simulink model "closed_loop_rider_PID"  (R2018b)
settings: Solver=VariableStepAuto  StartTime=0.0  StopTime=17.3  RelTol=1e-3
values from neighbouring files (symbols this model uses):
  G11_den = bike_s.Denominator{1, 1}    [data_analysis.m]
  G11_num = bike_s.Numerator{1, 1}    [data_analysis.m]
  G12_den = bike_s.Denominator{1, 2}    [data_analysis.m]
  G12_num = bike_s.Numerator{1, 2}    [data_analysis.m]
  G21_den = bike_s.Denominator{2, 1}    [data_analysis.m]
  G21_num = bike_s.Numerator{2, 1}    [data_analysis.m]
  G22_den = bike_s.Denominator{2, 2}    [data_analysis.m]
  G22_num = bike_s.Numerator{2, 2}    [data_analysis.m]
libraries: simulink x2
settings Model: Creator=chris  LastModifiedBy=chris

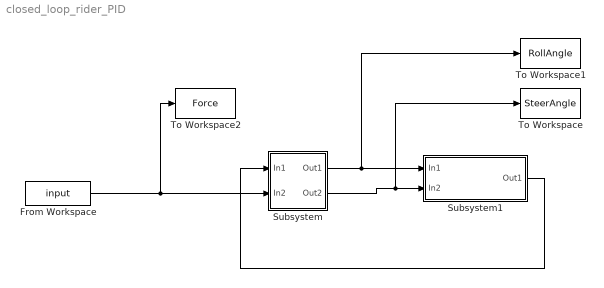
== system closed_loop_rider_PID ==
  From Workspace : FromWorkspace  VariableName=input  SampleTime=0
  Subsystem : Subsystem
  Subsystem1 : Subsystem
  To Workspace : ToWorkspace  VariableName=SteerAngle  SaveFormat=Timeseries  SampleTime=-1
  To Workspace1 : ToWorkspace  VariableName=RollAngle  SaveFormat=Timeseries  SampleTime=-1
  To Workspace2 : ToWorkspace  VariableName=Force  SaveFormat=Timeseries  SampleTime=-1
  wires:
  From Workspace/1 -> Subsystem/2(In2), To Workspace2/1
  Subsystem/1(Out1) -> To Workspace1/1, Subsystem1/1(In1)
  Subsystem1/1(Out1) -> Subsystem/1(In1)
  Subsystem/2(Out2) -> To Workspace/1, Subsystem1/2(In2)

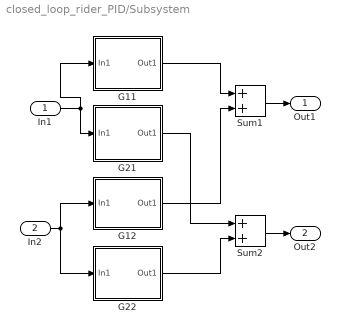
== system closed_loop_rider_PID/Subsystem ==
  In1 : Inport
  In2 : Inport  Port=2
  G11 : Subsystem
  G12 : Subsystem
  G21 : Subsystem
  G22 : Subsystem
  Sum1 : Sum  SaturateOnIntegerOverflow=on  InputSameDT=on  OutDataTypeStr=Inherit: Same as first input
  Sum2 : Sum  SaturateOnIntegerOverflow=on  InputSameDT=on  OutDataTypeStr=Inherit: Same as first input
  Out1 : Outport  InitialOutput=0
  Out2 : Outport  Port=2  InitialOutput=0
  wires:
  In1/1 -> G11/1(In1), G21/1(In1)
  G21/1(Out1) -> Sum2/1
  G12/1(Out1) -> Sum1/2
  G11/1(Out1) -> Sum1/1
  G22/1(Out1) -> Sum2/2
  In2/1 -> G12/1(In1), G22/1(In1)
  Sum1/1 -> Out1/1
  Sum2/1 -> Out2/1

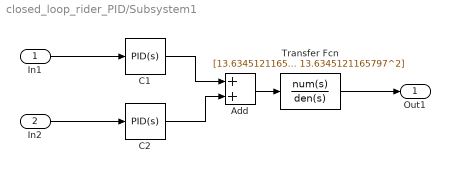
== system closed_loop_rider_PID/Subsystem1 ==
  In1 : Inport
  In2 : Inport  Port=2
  Add : Sum
  C1 : simulink/Continuous/PID Controller  Controller=PID  Form=Parallel  TimeDomain=Continuous-time  SampleTime=-1  IntegratorMethod=Forward Euler  FilterMethod=Forward Euler  ControllerParametersSource=internal  P=1  I=1  D=0  UseFilter=on  N=100  TunerSelectOption=Transfer Function Based (PID Tuner App)  InitialConditionSource=internal  InitialConditionForIntegrator=0  InitialConditionForFilter=0  DifferentiatorICPrevScaledInput=0  ExternalReset=none  TrackingMode=off  Kt=1  LimitOutput=off  UpperSaturationLimit=inf  LowerSaturationLimit=-inf  LinearizeAsGain=on  AntiWindupMode=none  Kb=1  POutMin=[]  POutMax=[]  IOutMin=[]  IOutMax=[]  DOutMin=[]  DOutMax=[]  NOutMin=[]  NOutMax=[]  SumOutMin=[]  SumOutMax=[]  SaturationOutMin=[]  SaturationOutMax=[]  PParamMin=[]  PParamMax=[]  IParamMin=[]  IParamMax=[]  DParamMin=[]  DParamMax=[]  NParamMin=[]  NParamMax=[]  KbParamMin=[]  KbParamMax=[]  KtParamMin=[]  KtParamMax=[]  KbOutMin=[]  KbOutMax=[]  KtOutMin=[]  KtOutMax=[]  IntegratorOutMin=[]  IntegratorOutMax=[]  FilterOutMin=[]  FilterOutMax=[]  SumI1OutMin=[]  SumI1OutMax=[]  SumI2OutMin=[]  SumI2OutMax=[]  SumI3OutMin=[]  SumI3OutMax=[]  SumI4OutMin=[]  SumI4OutMax=[]  SumDOutMin=[]  SumDOutMax=[]  DifferentiatorOutMin=[]  DifferentiatorOutMax=[]  FilterDiffOutCoefMin=[]  FilterDiffOutCoefMax=[]  ReciprocalOutMin=[]  ReciprocalOutMax=[]  SumDenOutMin=[]  SumDenOutMax=[]  SumNumOutMin=[]  SumNumOutMax=[]  DivideOutMin=[]  DivideOutMax=[]  IntegratorContinuousStateAttributes=''  IntegratorStateMustResolveToSignalObject=off  IntegratorRTWStateStorageClass=Auto  FilterContinuousStateAttributes=''  FilterStateMustResolveToSignalObject=off  FilterRTWStateStorageClass=Auto  ParallelPVariant=InternalParameters  IdealPVariant=Disabled  IVariant=InternalParameters  DVariant=InternalParameters  IntegratorVariant=Continuous  SatVariant=Disabled  AWVariant=Passthrough  PCopyVariant=Disabled  TRVariant=Disabled  FdbkBlocksVariant=Forward  IdealPFdbkVariant=Disabled  SatFdbkVariant=Disabled  DerivativeFilterVariant=ContFilter  NVariant=InternalParameters  NCopyVariant=Disabled  FilterICVariant=InternalICsFilter  IntegratorICVariant=InternalICs  ExternalResetVariant=Disabled  TRSumVariant=Passthrough  SumFdbkVariant=Disabled  SumVariant=Sum_PID
  C2 : simulink/Continuous/PID Controller  Controller=PID  Form=Parallel  TimeDomain=Continuous-time  SampleTime=-1  IntegratorMethod=Forward Euler  FilterMethod=Forward Euler  ControllerParametersSource=internal  P=1  I=1  D=0  UseFilter=on  N=100  TunerSelectOption=Transfer Function Based (PID Tuner App)  InitialConditionSource=internal  InitialConditionForIntegrator=0  InitialConditionForFilter=0  DifferentiatorICPrevScaledInput=0  ExternalReset=none  TrackingMode=off  Kt=1  LimitOutput=off  UpperSaturationLimit=inf  LowerSaturationLimit=-inf  LinearizeAsGain=on  AntiWindupMode=none  Kb=1  POutMin=[]  POutMax=[]  IOutMin=[]  IOutMax=[]  DOutMin=[]  DOutMax=[]  NOutMin=[]  NOutMax=[]  SumOutMin=[]  SumOutMax=[]  SaturationOutMin=[]  SaturationOutMax=[]  PParamMin=[]  PParamMax=[]  IParamMin=[]  IParamMax=[]  DParamMin=[]  DParamMax=[]  NParamMin=[]  NParamMax=[]  KbParamMin=[]  KbParamMax=[]  KtParamMin=[]  KtParamMax=[]  KbOutMin=[]  KbOutMax=[]  KtOutMin=[]  KtOutMax=[]  IntegratorOutMin=[]  IntegratorOutMax=[]  FilterOutMin=[]  FilterOutMax=[]  SumI1OutMin=[]  SumI1OutMax=[]  SumI2OutMin=[]  SumI2OutMax=[]  SumI3OutMin=[]  SumI3OutMax=[]  SumI4OutMin=[]  SumI4OutMax=[]  SumDOutMin=[]  SumDOutMax=[]  DifferentiatorOutMin=[]  DifferentiatorOutMax=[]  FilterDiffOutCoefMin=[]  FilterDiffOutCoefMax=[]  ReciprocalOutMin=[]  ReciprocalOutMax=[]  SumDenOutMin=[]  SumDenOutMax=[]  SumNumOutMin=[]  SumNumOutMax=[]  DivideOutMin=[]  DivideOutMax=[]  IntegratorContinuousStateAttributes=''  IntegratorStateMustResolveToSignalObject=off  IntegratorRTWStateStorageClass=Auto  FilterContinuousStateAttributes=''  FilterStateMustResolveToSignalObject=off  FilterRTWStateStorageClass=Auto  ParallelPVariant=InternalParameters  IdealPVariant=Disabled  IVariant=InternalParameters  DVariant=InternalParameters  IntegratorVariant=Continuous  SatVariant=Disabled  AWVariant=Passthrough  PCopyVariant=Disabled  TRVariant=Disabled  FdbkBlocksVariant=Forward  IdealPFdbkVariant=Disabled  SatFdbkVariant=Disabled  DerivativeFilterVariant=ContFilter  NVariant=InternalParameters  NCopyVariant=Disabled  FilterICVariant=InternalICsFilter  IntegratorICVariant=InternalICs  ExternalResetVariant=Disabled  TRSumVariant=Passthrough  SumFdbkVariant=Disabled  SumVariant=Sum_PID
  Transfer Fcn : TransferFcn  Numerator=[13.6345121165797^2]  Denominator=[1 19.2821119516073 13.6345121165797^2]
  Out1 : Outport
  wires:
  In1/1 -> C1/1
  C1/1 -> Add/1
  C2/1 -> Add/2
  In2/1 -> C2/1
  Add/1 -> Transfer Fcn/1
  Transfer Fcn/1 -> Out1/1

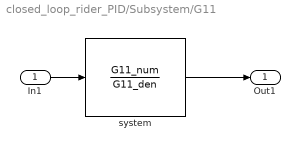
== system closed_loop_rider_PID/Subsystem/G11 ==
  In1 : Inport
  system : TransferFcn  Numerator=G11_num  Denominator=G11_den
  Out1 : Outport  InitialOutput=0
  wires:
  In1/1 -> system/1
  system/1 -> Out1/1

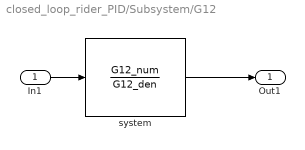
== system closed_loop_rider_PID/Subsystem/G12 ==
  In1 : Inport
  system : TransferFcn  Numerator=G12_num  Denominator=G12_den
  Out1 : Outport  InitialOutput=0
  wires:
  In1/1 -> system/1
  system/1 -> Out1/1

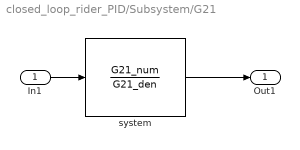
== system closed_loop_rider_PID/Subsystem/G21 ==
  In1 : Inport
  system : TransferFcn  Numerator=G21_num  Denominator=G21_den
  Out1 : Outport  InitialOutput=0
  wires:
  In1/1 -> system/1
  system/1 -> Out1/1

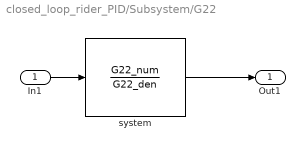
== system closed_loop_rider_PID/Subsystem/G22 ==
  In1 : Inport
  system : TransferFcn  Numerator=G22_num  Denominator=G22_den
  Out1 : Outport  InitialOutput=0
  wires:
  In1/1 -> system/1
  system/1 -> Out1/1
